simulink model "windaxes"  (Simulink 7.5)
settings: Solver=ode45  StartTime=0.0  StopTime=10.0  RelTol=1e-3
values from neighbouring files (symbols this model uses):
  a = b/0.246    (= 7.52032520325)    [valuables.m]
undefined symbols (not defined in the file or in its folder): tan2
settings Model: Creator=ex08148  LastModifiedBy=ex08148

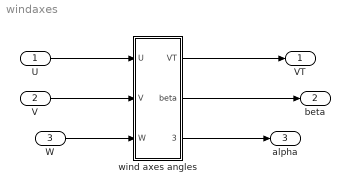
== system windaxes ==
  U : Inport  OutDataType=fixdt(1, 16)  OutScaling=2^0
  V : Inport  Port=2  OutDataType=fixdt(1, 16)  OutScaling=2^0
  W : Inport  Port=3  OutDataType=fixdt(1, 16)  OutScaling=2^0
  wind axes angles : Subsystem
  VT : Outport  OutDataType=fixdt(1, 16)  OutScaling=2^0
  beta : Outport  Port=2  OutDataType=fixdt(1, 16)  OutScaling=2^0
  alpha : Outport  Port=3  OutDataType=fixdt(1, 16)  OutScaling=2^0
  wires:
  U/1 -> wind axes angles/1(U)
  V/1 -> wind axes angles/2(V)
  wind axes angles/1(VT) -> VT/1
  W/1 -> wind axes angles/3(W)
  wind axes angles/2(beta) -> beta/1
  wind axes angles/3(alpha) -> alpha/1

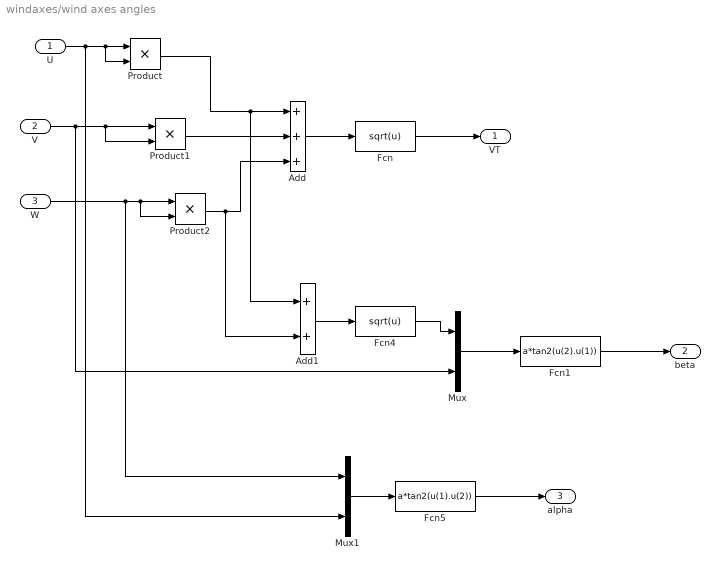
== system windaxes/wind axes angles ==
  U : Inport  OutDataType=fixdt(1, 16)  OutScaling=2^0
  V : Inport  Port=2  OutDataType=fixdt(1, 16)  OutScaling=2^0
  W : Inport  Port=3  OutDataType=fixdt(1, 16)  OutScaling=2^0
  Add : Sum  Inputs=+++  OutDataType=fixdt(1, 16)  OutScaling=2^-10
  Add1 : Sum  OutDataType=fixdt(1, 16)  OutScaling=2^-10
  Fcn : Fcn  Expr=sqrt(u)
  Fcn1 : Fcn  Expr=a*tan2(u(2).u(1))
  Fcn4 : Fcn  Expr=sqrt(u)
  Fcn5 : Fcn  Expr=a*tan2(u(1).u(2))
  Mux : Mux  Inputs=2
  Mux1 : Mux  Inputs=2
  Product : Product  OutDataType=fixdt(1, 16)  OutScaling=2^0  RndMeth=Zero
  Product1 : Product  OutDataType=fixdt(1, 16)  OutScaling=2^0  RndMeth=Zero
  Product2 : Product  OutDataType=fixdt(1, 16)  OutScaling=2^0  RndMeth=Zero
  VT : Outport  OutDataType=fixdt(1, 16)  OutScaling=2^0
  beta : Outport  Port=2  OutDataType=fixdt(1, 16)  OutScaling=2^0
  alpha : Outport  Port=3  OutDataType=fixdt(1, 16)  OutScaling=2^0
  wires:
  U/1 -> Product/1, Product/2, Mux1/2
  V/1 -> Product1/1, Product1/2, Mux/2
  W/1 -> Product2/1, Product2/2, Mux1/1
  Product/1 -> Add/1, Add1/1
  Product1/1 -> Add/2
  Product2/1 -> Add/3, Add1/2
  Add/1 -> Fcn/1
  Fcn/1 -> VT/1
  Add1/1 -> Fcn4/1
  Fcn4/1 -> Mux/1
  Mux/1 -> Fcn1/1
  Fcn1/1 -> beta/1
  Mux1/1 -> Fcn5/1
  Fcn5/1 -> alpha/1
